simulink model "demo4"  (Simulink 4.00)
settings: Solver=ode45  StartTime=0.0  StopTime=10.0  RelTol=1e-3
values from neighbouring files (symbols this model uses):
  p560 =     [matlab.mat]
undefined symbols (not defined in the file or in its folder): nofriction
libraries: roblocks x4, simulink3 x1
settings Model: Creator=pic  LastModifiedBy=pic  LimitDataPoints=off  ExtModeTrigMode=oneshot  ExtModeArmWhenConnect=off  BlockReductionOpt=off

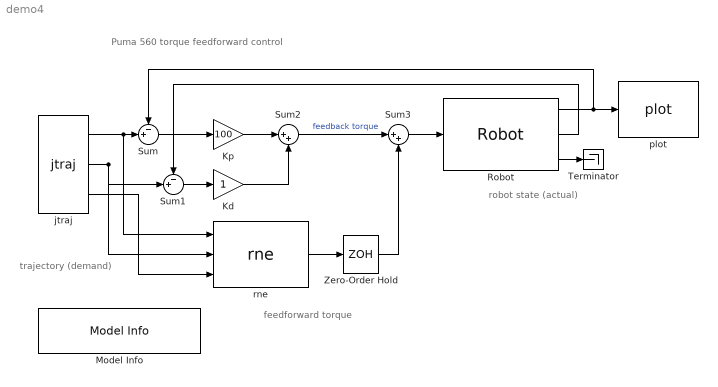
== system demo4 ==
  note: Puma 560 torque feedforward control
  note: trajectory
      | (demand)
  note: robot state
      | (actual)
  note: feedforward torque
  Kd : Gain  Gain=1  Multiplication=Element-wise(K.*u)  SaturateOnIntegerOverflow=on
  Kp : Gain  Gain=100  Multiplication=Element-wise(K.*u)  SaturateOnIntegerOverflow=on
  Model Info : simulink3/Signals & Systems/Model Info  InitialBlockCM=none  BlockCM=none  Frame=on  DisplayStringWithTags=|  HorizontalTextAlignment=Left  LeftAlignmentValue=0.02  SourceBlockDiagram=demo4  TagMaxNumber=20
      | Torque feedforward control
      | %<Creator>
      | %<LastModificationDate>
  Robot : roblocks/Robot  robot=nofriction(p560, 'coulomb')  q0=[0 0 0 0 0 0]
  Sum : Sum  Inputs=-+|  SaturateOnIntegerOverflow=on
  Sum1 : Sum  Inputs=-+|  SaturateOnIntegerOverflow=on
  Sum2 : Sum  Inputs=|++  SaturateOnIntegerOverflow=on
  Sum3 : Sum  Inputs=|++  SaturateOnIntegerOverflow=on
  Terminator : Terminator
  Zero-Order Hold : ZeroOrderHold  SampleTime=0.1
  jtraj : roblocks/jtraj  q0=[0 0 0 0 0 0]  qf=[pi/4 pi/2 -pi/2 0 0 0]  tmax=10
  plot : roblocks/plot  robot=p560
  rne : roblocks/rne  robot=nofriction(p560, 'coulomb')  grav=[0 0 9.81]
  wires:
  Kd/1 -> Sum2/2
  Sum/1 -> Kp/1
  Kp/1 -> Sum2/1
  Sum1/1 -> Kd/1
  Sum2/1 -> Sum3/1  "feedback torque"
  Sum3/1 -> Robot/1
  Robot/1 -> plot/1, Sum/1
  Robot/2 -> Sum1/1
  jtraj/1 -> Sum/2, rne/1
  jtraj/2 -> Sum1/2, rne/2
  Zero-Order Hold/1 -> Sum3/2
  rne/1 -> Zero-Order Hold/1
  jtraj/3 -> rne/3
  Robot/3 -> Terminator/1
